simulink model "MATLAB_TEST"  (R2019b)
settings: Solver=FixedStepDiscrete  StartTime=0  StopTime=50  FixedStep=0.0025  RelTol=1e-3
undefined symbols (not defined in the file): BCM_COM_PROC_P20, BCM_COM_PROC_P20_SFW_R2018b, BCM_COM_PROC_P2_5, BCM_COM_PROC_P2_5_SFW_R2018b, BCM_COM_PROC_P5, BCM_COM_PROC_P5_SFW_R2018b, BCMA_ACCU_PT_Conf_Flt, BCMA_ACCU_PT_Unconf_Flt, BCMA_Antiskid_Off_Sanction, BCMA_Avionics_Conf_Flt, BCMA_BCM_CCDL_Conf_Flt, BCMA_BCM_CCDL_Unconf_Flt, BCMA_BCM_DBCU_INHIBITION_Conf_Flt, BCMA_BCM_DBCU_INHIBITION_Unconf_Flt, BCMA_BCP_ALT_Disp_Sw_Conf_Flt, BCMA_BCP_ALT_Disp_Sw_Unconf_Flt, BCMA_BCP_ALT_SW_ON_CMD_Conf_Flt, BCMA_BCP_ALT_SW_ON_CMD_Unconf_Flt, BCMA_BCP_PARK_OFF_SW_CMD_Conf_Flt, BCMA_BCP_PARK_OFF_SW_CMD_Unconf_Flt, BCMA_CF_BSELV_JCL, BCMA_CF_BSELV_JOP, BCMA_CF_BSELV_OC, BCMA_CF_BSELV_SC, BCMA_CF_LH_SV_JCL, BCMA_CF_LH_SV_JOP, BCMA_CF_LH_SV_OC, BCMA_CF_LH_SV_SC, BCMA_CF_PARK_BRK, BCMA_CF_RESIDUAL_PRESS, BCMA_CF_RH_SV_JCL, BCMA_CF_RH_SV_JOP, BCMA_CF_RH_SV_OC, BCMA_CF_RH_SV_SC, BCMA_CF_SELV_JCL, BCMA_CF_SELV_JOP, BCMA_CF_SELV_OC, BCMA_CF_SELV_SC, BCMA_CF_SV_DRIFT, BCMA_DBCU_ALT_MODE_Conf_Flt, BCMA_DBCU_ALT_MODE_Unconf_Flt, BCMA_DBCU_BRK_ORDER_FAIL_Conf_Flt, BCMA_DBCU_BRK_ORDER_FAIL_Unconf_Flt, BCMA_DBCU_Conf_Flt, BCMA_DBCU_DISPATCH_SW_ON_Conf_Flt, BCMA_DBCU_DISPATCH_SW_ON_Unconf_Flt, BCMA_DBCU_FAILED_Conf_Flt, BCMA_DBCU_FAILED_Unconf_Flt, BCMA_DFCS1_Capsule_Validity, BCMA_DFCS1_Label202_Corrupted, BCMA_DFCS1_Label202_Not_Refreshed, BCMA_DFCS1_Label204_Corrupted, BCMA_DFCS1_Label204_Not_Refreshed, BCMA_DFCS1_Label205_Corrupted, BCMA_DFCS1_Label205_Not_Refreshed, BCMA_DFCS1_Label206_Corrupted, BCMA_DFCS1_Label206_Not_Refreshed, BCMA_DFCS1_Label207_Corrupted, BCMA_DFCS1_Label207_Not_Refreshed, BCMA_DFCS3_Capsule_Validity ... (+762)
libraries: simulink x73, lib_MBD_Control x5
(part 15 of 16)

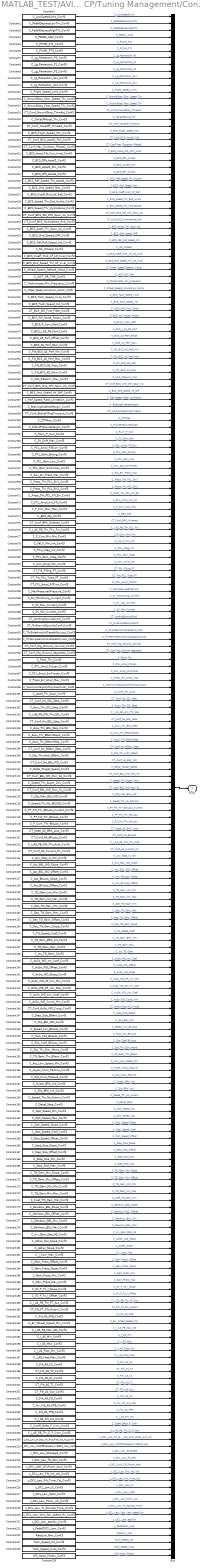
== system MATLAB_TEST/AVIONICS/Brake_Control_Module_Side_A/BCSA Controller CP/Tuning Management/Conf3 ==
  Bus : BusCreator  Inputs=226
  Constant1 : Constant  Value=C_LowSpeedLimit_Conf3
  Constant10 : Constant  Value=C_Lg_Retraction_SL1_Conf3
  Constant100 : Constant  Value=C_Accel_Thr_Auso_Conf3
  Constant101 : Constant  Value=CT_Conf_No_SSL_Step_Conf3
  Constant102 : Constant  Value=C_Accu_Thr_SSL_Step_Conf3
  Constant103 : Constant  Value=C_I_AS_PB_OW_Thr_SSL_Conf3
  Constant104 : Constant  Value=CT_Conf_No_BSL_Step_Conf3
  Constant105 : Constant  Value=C_Accu_Thr_BSL_Step_Conf3
  Constant106 : Constant  Value=C_Accu_Thr_BGamStep0_Conf3
  Constant107 : Constant  Value=C_Accu_Thr_BGamStep_Conf3
  Constant108 : Constant  Value=CT_Conf_No_BGam_Step_Conf3
  Constant109 : Constant  Value=C_Slip_Thr_Auth_BGam_Conf3
  Constant11 : Constant  Value=C_Lg_Retraction_SL2_Conf3
  Constant110 : Constant  Value=CT_Conf_No_BSL_WD_Conf3
  Constant111 : Constant  Value=C_Delta_Target_Speed_Conf3
  Constant112 : Constant  Value=CT_Conf_BSL_WD_Mon_FA_Conf3
  Constant113 : Constant  Value=C_Speed_Thr_Augm_Dim_Conf3
  Constant114 : Constant  Value=CT_Conf_BSL_WD_Mon_SL_Conf3
  Constant115 : Constant  Value=C_Slip_Max_BSL_WD_Conf3
  Constant116 : Constant  Value=C_Speed_Thr_No_BSLWD_Conf3
  Constant117 : Constant  Value=C_PT_Filt_Thr_BKLoss_Current_Conf3
  Constant118 : Constant  Value=C_PT_Filt_Thr_BKLoss_Conf3
  Constant119 : Constant  Value=C_P_Com_Thr_BKLoss_Conf3
  Constant12 : Constant  Value=C_Flight_Speed_Limit_Conf3
  Constant120 : Constant  Value=CT_Keep_AS_BRK_Loss_Conf3
  Constant121 : Constant  Value=CT_Conf_AS_BKLoss_Conf3
  Constant122 : Constant  Value=C_I_AS_PB_OW_Thr_Auth_Conf3
  Constant123 : Constant  Value=CT_Conf_AS_Current_On_Conf3
  Constant124 : Constant  Value=C_Any_Step_In_Min_Conf3
  Constant125 : Constant  Value=C_Acc_BSL_WD_Slope_Conf3
  Constant126 : Constant  Value=C_Acc_BSL_WD_Offset_Conf3
  Constant127 : Constant  Value=C_Acc_BKLoss_Slope_Conf3
  Constant128 : Constant  Value=C_Acc_BKLoss_Offset_Conf3
  Constant129 : Constant  Value=C_TG_Gam_Init_Min_Conf3
  Constant13 : Constant  Value=C_GroundStop_Slow_Speed_Thr_Conf3
  Constant130 : Constant  Value=C_TG_Gam_Init_Max_Conf3
  Constant131 : Constant  Value=C_Dec_TG_Gam_Min_Conf3
  Constant132 : Constant  Value=C_Dec_TG_Gam_Max_Conf3
  Constant133 : Constant  Value=C_Dec_TG_Gam_Offset_Conf3
  Constant134 : Constant  Value=C_Dec_TG_Gam_Slope_Conf3
  Constant135 : Constant  Value=C_TG_Speed_Coef_Conf3
  Constant136 : Constant  Value=C_TG_Gam_BRK_Init_Conf3
  Constant137 : Constant  Value=C_TG_Gam_Max_Conf3
  Constant138 : Constant  Value=C_Inc_TG_Gam_Conf3
  Constant139 : Constant  Value=C_AuSo_WD_Inc_Coef_Conf3
  Constant14 : Constant  Value=C_GroundStop_Fast_Speed_Thr_Conf3
  Constant140 : Constant  Value=C_AuSo_WD_Offset_Conf3
  Constant141 : Constant  Value=C_AuSo_WD_Slope_Conf3
  Constant142 : Constant  Value=C_AuSo_WD_SP_Lim_Min_Conf3
  Constant143 : Constant  Value=C_AuSo_WD_SP_Lim_Max_Conf3
  Constant144 : Constant  Value=C_AuSo_WD_Lim_Coef_Conf3
  Constant145 : Constant  Value=C_AuSo_WD_Count_Min_Conf3
  Constant146 : Constant  Value=CT_Conf_AuSo_WD_Froze_Conf3
  Constant147 : Constant  Value=C_Step_Size_BGam_Conf3
  Constant148 : Constant  Value=C_Slip_BSL_WD_Conf3
  Constant149 : Constant  Value=C_Speed_Lim_BKLoss_Conf3
  Constant15 : Constant  Value=CT_Conf_GroundStop_TimeAct_Conf3
  Constant150 : Constant  Value=C_Tach_Fail_BKLoss_Conf3
  Constant151 : Constant  Value=C_Slip_Coef_BKLoss_Conf3
  Constant152 : Constant  Value=C_Slip_Thr_Dim_Maint_Conf3
  Constant153 : Constant  Value=C_TG_Gam_Thr_BGam_Conf3
  Constant154 : Constant  Value=C_Acc_Low_Speed_Min_Conf3
  Constant155 : Constant  Value=C_Hyper_Cons_Passive_Conf3
  Constant156 : Constant  Value=C_Slip_Cons_Passive_Conf3
  Constant157 : Constant  Value=C_Hyper_BRK_Init_Conf3
  Constant158 : Constant  Value=C_Slip_BRK_Init_Conf3
  Constant159 : Constant  Value=C_Speed_Thr_No_Autom_Conf3
  Constant16 : Constant  Value=C_TakeOffAccel_Thr_Conf3
  Constant160 : Constant  Value=C_Decel_Step_Conf3
  Constant161 : Constant  Value=C_Opti_Speed_Min_Conf3
  Constant162 : Constant  Value=C_Opti_Speed_Max_Conf3
  Constant163 : Constant  Value=C_Opti_Speed_Slope_Conf3
  Constant164 : Constant  Value=C_Opti_Speed_Coef_Conf3
  Constant165 : Constant  Value=C_Opti_Speed_Offset_Conf3
  Constant166 : Constant  Value=C_Step_Size_Slope_Conf3
  Constant167 : Constant  Value=C_Step_Size_Offset_Conf3
  Constant168 : Constant  Value=C_Step_Size_Min_Conf3
  Constant169 : Constant  Value=C_Step_Size_Max_Conf3
  Constant17 : Constant  Value=CT_Conf_TakeOff_TimeAct_Conf3
  Constant170 : Constant  Value=C_TG_Gam_Min_Slope_Conf3
  Constant171 : Constant  Value=C_TG_Gam_Min_Offset_Conf3
  Constant172 : Constant  Value=C_TG_Gam_Min_Min_Conf3
  Constant173 : Constant  Value=C_TG_Gam_Min_Max_Conf3
  Constant174 : Constant  Value=C_Coef_TG_Gam_Min_Conf3
  Constant175 : Constant  Value=C_DenAccu_BSL_Slope_Conf3
  Constant176 : Constant  Value=C_DenAccu_BSL_Offset_Conf3
  Constant177 : Constant  Value=C_DenAccu_BSL_Min_Conf3
  Constant178 : Constant  Value=C_DenAccu_BSL_Max_Conf3
  Constant179 : Constant  Value=C_Inv_Gain_Stat_AS_Conf3
  Constant18 : Constant  Value=C_BCS_Flight_Speed_Min_Conf3
  Constant180 : Constant  Value=C_Adher_Opt_Slope_Conf3
  Constant181 : Constant  Value=C_Adher_Slope_Conf3
  Constant182 : Constant  Value=C_I_Com_Max_Conf3
  Constant183 : Constant  Value=C_Gain_Press_Offset_Conf3
  Constant184 : Constant  Value=C_Gain_Press_Slope_Conf3
  Constant185 : Constant  Value=C_Gain_Press_Min_Conf3
  Constant186 : Constant  Value=C_Gain_Press_Max_Conf3
  Constant187 : Constant  Value=C_SV_P_To_I_Slope_Conf3
  Constant188 : Constant  Value=C_SV_P_To_I_Offset_Conf3
  Constant189 : Constant  Value=C_I_AS_PB_Thr_PT_Aut_Conf3
  Constant19 : Constant  Value=CT_Conf_BCS_Accel2_Fail_Conf3
  Constant190 : Constant  Value=CT_Filt_PT_Filt_Autom_Conf3
  Constant191 : Constant  Value=C_Filt_AS_KPB_Conf3
  Constant192 : Constant  Value=C_Err_Wheel_Speed_Min_Conf3
  Constant193 : Constant  Value=C_I_AS_PB_Max_ND_Conf3
  Constant194 : Constant  Value=C_I_AS_Min_Conf3
  Constant195 : Constant  Value=C_I_AS_Max_Conf3
  Constant196 : Constant  Value=C_I_AS_Fast_Min_Conf3
  Constant197 : Constant  Value=C_I_AS_Fast_Max_Conf3
  Constant198 : Constant  Value=C_Filt_AS_K2_Conf3
  Constant199 : Constant  Value=CT_Filt_AS_T2_Conf3
  Constant2 : Constant  Value=C_PedalDepressLowThr_Conf3
  Constant20 : Constant  Value=CT_Conf_Max_Duration_Phase2_Conf3
  Constant200 : Constant  Value=C_Filt_AS_K1_Conf3
  Constant201 : Constant  Value=CT_Filt_AS_T1_Conf3
  Constant202 : Constant  Value=CT_Filt_AS_Out_Conf3
  Constant203 : Constant  Value=C_Filt_AS_K0_Conf3
  Constant204 : Constant  Value=C_Inv_Filt_AS_KPB_Conf3
  Constant205 : Constant  Value=C_Filt_AS_TPB_Conf3
  Constant206 : Constant  Value=C_I_AS_Filt_Init_Conf3
  Constant207 : Constant  Value=C_Coeff_Delta_P_Com_Conf3
  Constant208 : Constant  Value=C_I_AS_PB_Thr_D_P_Com_Conf3
  Constant209 : Constant  Value=c_DCL_Law_CT_BCS_WS_First_Filter_Acc_AC_Conf3
  Constant21 : Constant  Value=C_BCS_Accel_Filt_Corr_Inval_Conf3
  Constant210 : Constant  Value=c_DCL_Law_CutOffFrequencyVSGRS_Law_Conf3
  Constant211 : Constant  Value=c_DCL_Law_Strategie_Conf3
  Constant212 : Constant  Value=c_DCL_Law_filt_8Hz_Conf3
  Constant213 : Constant  Value=c_DCL_LAW_DCLPcom_bool_Conf3
  Constant214 : Constant  Value=c_DCL_Law_Filt_Init_Val_Conf3
  Constant215 : Constant  Value=c_DCL_Law_Filt_Time_Cst_Conf3
  Constant216 : Constant  Value=c_DCL_Law_Ki_Conf3
  Constant217 : Constant  Value=c_DCL_Law_Kpb2_Conf3
  Constant218 : Constant  Value=c_DCL_Law_Pcom_var_Conf3
  Constant219 : Constant  Value=c_DCL_Law_Ts_Sample_Time_Conf3
  Constant22 : Constant  Value=C_BCS_Dflt_Accel2_Conf3
  Constant220 : Constant  Value=c_DCL_Law_Very_law_speed_thr_Conf3
  Constant221 : Constant  Value=c_DCL_Law_epsilon_Conf3
  Constant222 : Constant  Value=c_Pedal2DCL_Law_Conf3
  Constant223 : Constant  Value=RateLim_Max_Conf3
  Constant224 : Constant  Value=Tach_Speed_Init_Conf3
  Constant225 : Constant  Value=Tach_Speed_Inval_Conf3
  Constant226 : Constant  Value=WS_Noise_Factor_Conf3
  Constant23 : Constant  Value=C_BCS_Accel3_Min_Conf3
  Constant24 : Constant  Value=C_BCS_Dflt_Accel4_Conf3
  Constant25 : Constant  Value=C_BCS_Ref_Speed_Thr_Accel4_Conf3
  Constant26 : Constant  Value=C_BCS_Gnd_Speed_Max_Conf3
  Constant27 : Constant  Value=C_BCS_Coeff_Mult_Inf_Ref_Conf3
  Constant28 : Constant  Value=C_BCS_Speed_Thr_End_Hydro_Conf3
  Constant29 : Constant  Value=C_BCS_Speed_Thr_Hydroplane_Conf3
  Constant3 : Constant  Value=C_PedalDepressHighThr_Conf3
  Constant30 : Constant  Value=CT_Conf_BCS_Gbl_Whl_Spun_Up_Conf3
  Constant31 : Constant  Value=CT_Conf_BCS_Hydroplane_End_Conf3
  Constant32 : Constant  Value=C_BCS_Accel_Thr_Spun_Up_Conf3
  Constant33 : Constant  Value=C_BCS_Gnd_Speed_Diff_Conf3
  Constant34 : Constant  Value=C_BCS_Gbl_Ref_Speed_Init_Conf3
  Constant35 : Constant  Value=C_Nb_Wheels_Conf3
  Constant36 : Constant  Value=C_BCS_Coeff_Mult_Inf_LG_Inval_Conf3
  Constant37 : Constant  Value=C_BCS_Gnd_Speed_Thr_LG_Inval_Conf3
  Constant38 : Constant  Value=C_Wheel_Speed_Default_Value_Conf3
  Constant39 : Constant  Value=C_WST_OR_THR_Conf3
  Constant4 : Constant  Value=C_PEDAL_LAW_Conf3
  Constant40 : Constant  Value=C_Tachometer_Min_Frequency_Conf3
  Constant41 : Constant  Value=C_Wheel_Speed_Conversion_Factor_Conf3
  Constant42 : Constant  Value=C_BCS_Tach_Speed_Inval_Conf3
  Constant43 : Constant  Value=C_BCS_Tach_Speed_Init_Conf3
  Constant44 : Constant  Value=CT_BCS_WS_First_Filter_Conf3
  Constant45 : Constant  Value=C_BCS_WS_Noise_Factor_Conf3
  Constant46 : Constant  Value=C_BCS_P_Com_Perf_Conf3
  Constant47 : Constant  Value=C_BCS_I_AS_PB_Perf_Conf3
  Constant48 : Constant  Value=C_BCS_AS_Perf_Offset_Conf3
  Constant49 : Constant  Value=C_BCS_AS_Perf_Gain_Conf3
  Constant5 : Constant  Value=C_PCOM_FT1_Conf3
  Constant50 : Constant  Value=C_Filt_BCS_AS_Perf_Min_Conf3
  Constant51 : Constant  Value=C_Filt_BCS_AS_Perf_Max_Conf3
  Constant52 : Constant  Value=C_Filt_BCS_AS_Fast_Conf3
  Constant53 : Constant  Value=C_Filt_BCS_AS_Slow_Conf3
  Constant54 : Constant  Value=C_Wst_RateLim_Max_Conf3
  Constant55 : Constant  Value=CT_Conf_BCS_One_Whl_Spun_Up_Conf3
  Constant56 : Constant  Value=C_BCS_Gnd_Speed_Inf_Diff_Conf3
  Constant57 : Constant  Value=C_Ref_Speed_Rate_Limitation_Conf3
  Constant58 : Constant  Value=C_BrakingOrderedMargin_Conf3
  Constant59 : Constant  Value=CT_Conf_BrakeFillingTimeout_Conf3
  Constant6 : Constant  Value=C_PCOM_FT3_Conf3
  Constant60 : Constant  Value=C_ZTPMax_Conf3
  Constant61 : Constant  Value=C_FilloutPressureMargin_Conf3
  Constant62 : Constant  Value=C_RLim_P_Corr_Conf3
  Constant63 : Constant  Value=C_SV_Drift_Max_Conf3
  Constant64 : Constant  Value=C_PCL_Ampl_FillCorr_Conf3
  Constant65 : Constant  Value=C_PCL_Gain_Strong_Conf3
  Constant66 : Constant  Value=C_PCL_Gain_Low_Conf3
  Constant67 : Constant  Value=C_PCL_Gain_SmFrozen_Conf3
  Constant68 : Constant  Value=C_Squ_Err_Press_Max_Conf3
  Constant69 : Constant  Value=C_Press_Thr_PCL_Err1_Conf3
  Constant7 : Constant  Value=C_Lg_Retraction_P0_Conf3
  Constant70 : Constant  Value=C_Press_Thr_PCL_Err2_Conf3
  Constant71 : Constant  Value=C_Press_Thr_PCL_Fill_Err_Conf3
  Constant72 : Constant  Value=C_PCL_Ampl_Init_Fill_Conf3
  Constant73 : Constant  Value=C_P_Corr_Max_Max_Conf3
  Constant74 : Constant  Value=C_BCS_Ztp_Conf3
  Constant75 : Constant  Value=CT_Conf_BRK_Ordered_Conf3
  Constant76 : Constant  Value=C_I_AS_PB_Thr_PCL_Frz_Conf3
  Constant77 : Constant  Value=C_P_Corr_Min_Min_Conf3
  Constant78 : Constant  Value=C_Val_P_Min_Init_Conf3
  Constant79 : Constant  Value=C_PCL_Integ_Init_Conf3
  Constant8 : Constant  Value=C_Lg_Retraction_P1_Conf3
  Constant80 : Constant  Value=C_PCL_Gain_Integ_Conf3
  Constant81 : Constant  Value=C_Corr_Ampl_Min_Conf3
  Constant82 : Constant  Value=CT_Filt_Filling_PT_Conf3
  Constant83 : Constant  Value=CT_Filt_PCL_Tube_PT_Conf3
  Constant84 : Constant  Value=CT_PCL_Ampl_FillCorr_Conf3
  Constant85 : Constant  Value=C_MaxMeasuredPressure_Conf3
  Constant86 : Constant  Value=C_SV_Monitoring_Current_Conf3
  Constant87 : Constant  Value=C_SV_Max_Current_Conf3
  Constant88 : Constant  Value=C_SV_Min_Current_Conf3
  Constant89 : Constant  Value=CT_LandingSpunUpConf_Conf3
  Constant9 : Constant  Value=C_Lg_Retraction_P2_Conf3
  Constant90 : Constant  Value=CT_OnGroundSpunUpConf_Conf3
  Constant91 : Constant  Value=C_ThrSideAntiskidCapabilityLoss_Conf3
  Constant92 : Constant  Value=C_ThrPerimeterAntiskidCapabilityLoss_Conf3
  Constant93 : Constant  Value=CT_Conf_Nlg_Ground_nominal_Conf3
  Constant94 : Constant  Value=CT_Conf_Nlg_Ground_degraded_Conf3
  Constant95 : Constant  Value=C_Pitch_Thr_Conf3
  Constant96 : Constant  Value=C_PCL_Ampl_Frozen_Conf3
  Constant97 : Constant  Value=C_PCL_Ampl_SmFrozen_Conf3
  Constant98 : Constant  Value=C_Press_Err_Ampl_Max_Conf3
  Constant99 : Constant  Value=C_MaximumMarginWithHydraulicLost_Conf3
  Out1 : Outport  VectorParamsAs1DForOutWhenUnconnected=off
  wires:
  Constant1/1 -> Bus/1  "C_LowSpeedLimit"
  Constant2/1 -> Bus/2  "C_PedalDepressLowThr"
  Constant3/1 -> Bus/3  "C_PedalDepressHighThr"
  Constant4/1 -> Bus/4  "C_PEDAL_LAW"
  Constant5/1 -> Bus/5  "C_PCOM_FT1"
  Constant6/1 -> Bus/6  "C_PCOM_FT3"
  Constant7/1 -> Bus/7  "C_Lg_Retraction_P0"
  Constant8/1 -> Bus/8  "C_Lg_Retraction_P1"
  Constant9/1 -> Bus/9  "C_Lg_Retraction_P2"
  Constant10/1 -> Bus/10  "C_Lg_Retraction_SL1"
  Constant11/1 -> Bus/11  "C_Lg_Retraction_SL2"
  Constant12/1 -> Bus/12  "C_Flight_Speed_Limit"
  Constant13/1 -> Bus/13  "C_GroundStop_Slow_Speed_Thr"
  Constant14/1 -> Bus/14  "C_GroundStop_Fast_Speed_Thr"
  Constant15/1 -> Bus/15  "CT_Conf_GroundStop_TimeAct"
  Constant16/1 -> Bus/16  "C_TakeOffAccel_Thr"
  Constant17/1 -> Bus/17  "CT_Conf_TakeOff_TimeAct"
  Constant18/1 -> Bus/18  "C_BCS_Flight_Speed_Min"
  Constant19/1 -> Bus/19  "CT_Conf_BCS_Accel2_Fail"
  Constant20/1 -> Bus/20  "CT_Conf_Max_Duration_Phase2"
  Constant21/1 -> Bus/21  "C_BCS_Accel_Filt_Corr_Inval"
  Constant22/1 -> Bus/22  "C_BCS_Dflt_Accel2"
  Constant23/1 -> Bus/23  "C_BCS_Accel3_Min"
  Constant24/1 -> Bus/24  "C_BCS_Dflt_Accel4"
  Constant25/1 -> Bus/25  "C_BCS_Ref_Speed_Thr_Accel4"
  Constant26/1 -> Bus/26  "C_BCS_Gnd_Speed_Max"
  Constant27/1 -> Bus/27  "C_BCS_Coeff_Mult_Inf_Ref"
  Constant28/1 -> Bus/28  "C_BCS_Speed_Thr_End_Hydro"
  Constant29/1 -> Bus/29  "C_BCS_Speed_Thr_Hydroplane"
  Constant30/1 -> Bus/30  "CT_Conf_BCS_Gbl_Whl_Spun_Up"
  Constant31/1 -> Bus/31  "CT_Conf_BCS_Hydroplane_End"
  Constant32/1 -> Bus/32  "C_BCS_Accel_Thr_Spun_Up"
  Constant33/1 -> Bus/33  "C_BCS_Gnd_Speed_Diff"
  Constant34/1 -> Bus/34  "C_BCS_Gbl_Ref_Speed_Init"
  Constant35/1 -> Bus/35  "C_Nb_Wheels"
  Constant36/1 -> Bus/36  "C_BCS_Coeff_Mult_Inf_LG_Inval"
  Constant37/1 -> Bus/37  "C_BCS_Gnd_Speed_Thr_LG_Inval"
  Constant38/1 -> Bus/38  "C_Wheel_Speed_Default_Value"
  Constant39/1 -> Bus/39  "C_WST_OR_THR"
  Constant40/1 -> Bus/40  "C_Tachometer_Min_Frequency"
  Constant41/1 -> Bus/41  "C_Wheel_Speed_Conversion_Factor"
  Constant42/1 -> Bus/42  "C_BCS_Tach_Speed_Inval"
  Constant43/1 -> Bus/43  "C_BCS_Tach_Speed_Init"
  Constant44/1 -> Bus/44  "CT_BCS_WS_First_Filter"
  Constant45/1 -> Bus/45  "C_BCS_WS_Noise_Factor"
  Constant46/1 -> Bus/46  "C_BCS_P_Com_Perf"
  Constant47/1 -> Bus/47  "C_BCS_I_AS_PB_Perf"
  Constant48/1 -> Bus/48  "C_BCS_AS_Perf_Offset"
  Constant49/1 -> Bus/49  "C_BCS_AS_Perf_Gain"
  Constant50/1 -> Bus/50  "C_Filt_BCS_AS_Perf_Min"
  Constant51/1 -> Bus/51  "C_Filt_BCS_AS_Perf_Max"
  Constant52/1 -> Bus/52  "C_Filt_BCS_AS_Fast"
  Constant53/1 -> Bus/53  "C_Filt_BCS_AS_Slow"
  Constant54/1 -> Bus/54  "C_Wst_RateLim_Max"
  Constant55/1 -> Bus/55  "CT_Conf_BCS_One_Whl_Spun_Up"
  Constant56/1 -> Bus/56  "C_BCS_Gnd_Speed_Inf_Diff"
  Constant57/1 -> Bus/57  "C_Ref_Speed_Rate_Limitation"
  Constant58/1 -> Bus/58  "C_BrakingOrderedMargin"
  Constant59/1 -> Bus/59  "CT_Conf_BrakeFillingTimeout"
  Constant60/1 -> Bus/60  "C_ZTPMax"
  Constant61/1 -> Bus/61  "C_FilloutPressureMargin"
  Constant62/1 -> Bus/62  "C_RLim_P_Corr"
  Constant63/1 -> Bus/63  "C_SV_Drift_Max"
  Constant64/1 -> Bus/64  "C_PCL_Ampl_FillCorr"
  Constant65/1 -> Bus/65  "C_PCL_Gain_Strong"
  Constant66/1 -> Bus/66  "C_PCL_Gain_Low"
  Constant67/1 -> Bus/67  "C_PCL_Gain_SmFrozen"
  Constant68/1 -> Bus/68  "C_Squ_Err_Press_Max"
  Constant69/1 -> Bus/69  "C_Press_Thr_PCL_Err1"
  Constant70/1 -> Bus/70  "C_Press_Thr_PCL_Err2"
  Constant71/1 -> Bus/71  "C_Press_Thr_PCL_Fill_Err"
  Constant72/1 -> Bus/72  "C_PCL_Ampl_Init_Fill"
  Constant73/1 -> Bus/73  "C_P_Corr_Max_Max"
  Constant74/1 -> Bus/74  "C_BCS_Ztp"
  Constant75/1 -> Bus/75  "CT_Conf_BRK_Ordered"
  Constant76/1 -> Bus/76  "C_I_AS_PB_Thr_PCL_Frz"
  Constant77/1 -> Bus/77  "C_P_Corr_Min_Min"
  Constant78/1 -> Bus/78  "C_Val_P_Min_Init"
  Constant79/1 -> Bus/79  "C_PCL_Integ_Init"
  Constant80/1 -> Bus/80  "C_PCL_Gain_Integ"
  Constant81/1 -> Bus/81  "C_Corr_Ampl_Min"
  Constant82/1 -> Bus/82  "CT_Filt_Filling_PT"
  Constant83/1 -> Bus/83  "CT_Filt_PCL_Tube_PT"
  Constant84/1 -> Bus/84  "CT_PCL_Ampl_FillCorr"
  Constant85/1 -> Bus/85  "C_MaxMeasuredPressure"
  Constant86/1 -> Bus/86  "C_SV_Monitoring_Current"
  Constant87/1 -> Bus/87  "C_SV_Max_Current"
  Constant88/1 -> Bus/88  "C_SV_Min_Current"
  Constant89/1 -> Bus/89  "CT_LandingSpunUpConf"
  Constant90/1 -> Bus/90  "CT_OnGroundSpunUpConf"
  Constant91/1 -> Bus/91  "C_ThrSideAntiskidCapabilityLoss"
  Constant92/1 -> Bus/92  "C_ThrPerimeterAntiskidCapabilityLoss"
  Constant93/1 -> Bus/93  "CT_Conf_Nlg_Ground_nominal"
  Constant94/1 -> Bus/94  "CT_Conf_Nlg_Ground_degraded"
  Constant95/1 -> Bus/95  "C_Pitch_Thr"
  Constant96/1 -> Bus/96  "C_PCL_Ampl_Frozen"
  Constant97/1 -> Bus/97  "C_PCL_Ampl_SmFrozen"
  Constant98/1 -> Bus/98  "C_Press_Err_Ampl_Max"
  Constant99/1 -> Bus/99  "C_MaximumMarginWithHydraulicLost"
  Constant100/1 -> Bus/100  "C_Accel_Thr_Auso"
  Constant101/1 -> Bus/101  "CT_Conf_No_SSL_Step"
  Constant102/1 -> Bus/102  "C_Accu_Thr_SSL_Step"
  Constant103/1 -> Bus/103  "C_I_AS_PB_OW_Thr_SSL"
  Constant104/1 -> Bus/104  "CT_Conf_No_BSL_Step"
  Constant105/1 -> Bus/105  "C_Accu_Thr_BSL_Step"
  Constant106/1 -> Bus/106  "C_Accu_Thr_BGamStep0"
  Constant107/1 -> Bus/107  "C_Accu_Thr_BGamStep"
  Constant108/1 -> Bus/108  "CT_Conf_No_BGam_Step"
  Constant109/1 -> Bus/109  "C_Slip_Thr_Auth_BGam"
  Constant110/1 -> Bus/110  "CT_Conf_No_BSL_WD"
  Constant111/1 -> Bus/111  "C_Delta_Target_Speed"
  Constant112/1 -> Bus/112  "CT_Conf_BSL_WD_Mon_FA"
  Constant113/1 -> Bus/113  "C_Speed_Thr_Augm_Dim"
  Constant114/1 -> Bus/114  "CT_Conf_BSL_WD_Mon_SL"
  Constant115/1 -> Bus/115  "C_Slip_Max_BSL_WD"
  Constant116/1 -> Bus/116  "C_Speed_Thr_No_BSLWD"
  Constant117/1 -> Bus/117  "C_PT_Filt_Thr_BKLoss_Current"
  Constant118/1 -> Bus/118  "C_PT_Filt_Thr_BKLoss"
  Constant119/1 -> Bus/119  "C_P_Com_Thr_BKLoss"
  Constant120/1 -> Bus/120  "CT_Keep_AS_BRK_Loss"
  Constant121/1 -> Bus/121  "CT_Conf_AS_BKLoss"
  Constant122/1 -> Bus/122  "C_I_AS_PB_OW_Thr_Auth"
  Constant123/1 -> Bus/123  "CT_Conf_AS_Current_On"
  Constant124/1 -> Bus/124  "C_Any_Step_In_Min"
  Constant125/1 -> Bus/125  "C_Acc_BSL_WD_Slope"
  Constant126/1 -> Bus/126  "C_Acc_BSL_WD_Offset"
  Constant127/1 -> Bus/127  "C_Acc_BKLoss_Slope"
  Constant128/1 -> Bus/128  "C_Acc_BKLoss_Offset"
  Constant129/1 -> Bus/129  "C_TG_Gam_Init_Min"
  Constant130/1 -> Bus/130  "C_TG_Gam_Init_Max"
  Constant131/1 -> Bus/131  "C_Dec_TG_Gam_Min"
  Constant132/1 -> Bus/132  "C_Dec_TG_Gam_Max"
  Constant133/1 -> Bus/133  "C_Dec_TG_Gam_Offset"
  Constant134/1 -> Bus/134  "C_Dec_TG_Gam_Slope"
  Constant135/1 -> Bus/135  "C_TG_Speed_Coef"
  Constant136/1 -> Bus/136  "C_TG_Gam_BRK_Init"
  Constant137/1 -> Bus/137  "C_TG_Gam_Max"
  Constant138/1 -> Bus/138  "C_Inc_TG_Gam"
  Constant139/1 -> Bus/139  "C_AuSo_WD_Inc_Coef"
  Constant140/1 -> Bus/140  "C_AuSo_WD_Offset"
  Constant141/1 -> Bus/141  "C_AuSo_WD_Slope"
  Constant142/1 -> Bus/142  "C_AuSo_WD_SP_Lim_Min"
  Constant143/1 -> Bus/143  "C_AuSo_WD_SP_Lim_Max"
  Constant144/1 -> Bus/144  "C_AuSo_WD_Lim_Coef"
  Constant145/1 -> Bus/145  "C_AuSo_WD_Count_Min"
  Constant146/1 -> Bus/146  "CT_Conf_AuSo_WD_Froze"
  Constant147/1 -> Bus/147  "C_Step_Size_BGam"
  Constant148/1 -> Bus/148  "C_Slip_BSL_WD"
  Constant149/1 -> Bus/149  "C_Speed_Lim_BKLoss"
  Constant150/1 -> Bus/150  "C_Tach_Fail_BKLoss"
  Constant151/1 -> Bus/151  "C_Slip_Coef_BKLoss"
  Constant152/1 -> Bus/152  "C_Slip_Thr_Dim_Maint"
  Constant153/1 -> Bus/153  "C_TG_Gam_Thr_BGam"
  Constant154/1 -> Bus/154  "C_Acc_Low_Speed_Min"
  Constant155/1 -> Bus/155  "C_Hyper_Cons_Passive"
  Constant156/1 -> Bus/156  "C_Slip_Cons_Passive"
  Constant157/1 -> Bus/157  "C_Hyper_BRK_Init"
  Constant158/1 -> Bus/158  "C_Slip_BRK_Init"
  Constant159/1 -> Bus/159  "C_Speed_Thr_No_Autom"
  Constant160/1 -> Bus/160  "C_Decel_Step"
  Constant161/1 -> Bus/161  "C_Opti_Speed_Min"
  Constant162/1 -> Bus/162  "C_Opti_Speed_Max"
  Constant163/1 -> Bus/163  "C_Opti_Speed_Slope"
  Constant164/1 -> Bus/164  "C_Opti_Speed_Coef"
  Constant165/1 -> Bus/165  "C_Opti_Speed_Offset"
  Constant166/1 -> Bus/166  "C_Step_Size_Slope"
  Constant167/1 -> Bus/167  "C_Step_Size_Offset"
  Constant168/1 -> Bus/168  "C_Step_Size_Min"
  Constant169/1 -> Bus/169  "C_Step_Size_Max"
  Constant170/1 -> Bus/170  "C_TG_Gam_Min_Slope"
  Constant171/1 -> Bus/171  "C_TG_Gam_Min_Offset"
  Constant172/1 -> Bus/172  "C_TG_Gam_Min_Min"
  Constant173/1 -> Bus/173  "C_TG_Gam_Min_Max"
  Constant174/1 -> Bus/174  "C_Coef_TG_Gam_Min"
  Constant175/1 -> Bus/175  "C_DenAccu_BSL_Slope"
  Constant176/1 -> Bus/176  "C_DenAccu_BSL_Offset"
  Constant177/1 -> Bus/177  "C_DenAccu_BSL_Min"
  Constant178/1 -> Bus/178  "C_DenAccu_BSL_Max"
  Constant179/1 -> Bus/179  "C_Inv_Gain_Stat_AS"
  Constant180/1 -> Bus/180  "C_Adher_Opt_Slope"
  Constant181/1 -> Bus/181  "C_Adher_Slope"
  Constant182/1 -> Bus/182  "C_I_Com_Max"
  Constant183/1 -> Bus/183  "C_Gain_Press_Offset"
  Constant184/1 -> Bus/184  "C_Gain_Press_Slope"
  Constant185/1 -> Bus/185  "C_Gain_Press_Min"
  Constant186/1 -> Bus/186  "C_Gain_Press_Max"
  Constant187/1 -> Bus/187  "C_SV_P_To_I_Slope"
  Constant188/1 -> Bus/188  "C_SV_P_To_I_Offset"
  Constant189/1 -> Bus/189  "C_I_AS_PB_Thr_PT_Aut"
  Constant190/1 -> Bus/190  "CT_Filt_PT_Filt_Autom"
  Constant191/1 -> Bus/191  "C_Filt_AS_KPB"
  Constant192/1 -> Bus/192  "C_Err_Wheel_Speed_Min"
  Constant193/1 -> Bus/193  "C_I_AS_PB_Max_ND"
  Constant194/1 -> Bus/194  "C_I_AS_Min"
  Constant195/1 -> Bus/195  "C_I_AS_Max"
  Constant196/1 -> Bus/196  "C_I_AS_Fast_Min"
  Constant197/1 -> Bus/197  "C_I_AS_Fast_Max"
  Constant198/1 -> Bus/198  "C_Filt_AS_K2"
  Constant199/1 -> Bus/199  "CT_Filt_AS_T2"
  Constant200/1 -> Bus/200  "C_Filt_AS_K1"
  Constant201/1 -> Bus/201  "CT_Filt_AS_T1"
  Constant202/1 -> Bus/202  "CT_Filt_AS_Out"
  Constant203/1 -> Bus/203  "C_Filt_AS_K0"
  Constant204/1 -> Bus/204  "C_Inv_Filt_AS_KPB"
  Constant205/1 -> Bus/205  "C_Filt_AS_TPB"
  Constant206/1 -> Bus/206  "C_I_AS_Filt_Init"
  Constant207/1 -> Bus/207  "C_Coeff_Delta_P_Com"
  Constant208/1 -> Bus/208  "C_I_AS_PB_Thr_D_P_Com"
  Constant209/1 -> Bus/209  "c_DCL_Law_CT_BCS_WS_First_Filter_Acc_AC"
  Constant210/1 -> Bus/210  "c_DCL_Law_CutOffFrequencyVSGRS_Law"
  Constant211/1 -> Bus/211  "c_DCL_Law_Strategie"
  Constant212/1 -> Bus/212  "c_DCL_Law_filt_8Hz"
  Constant213/1 -> Bus/213  "c_DCL_LAW_DCLPcom_bool"
  Constant214/1 -> Bus/214  "c_DCL_Law_Filt_Init_Val"
  Constant215/1 -> Bus/215  "c_DCL_Law_Filt_Time_Cst"
  Constant216/1 -> Bus/216  "c_DCL_Law_Ki"
  Constant217/1 -> Bus/217  "c_DCL_Law_Kpb2"
  Constant218/1 -> Bus/218  "c_DCL_Law_Pcom_var"
  Constant219/1 -> Bus/219  "c_DCL_Law_Ts_Sample_Time"
  Constant220/1 -> Bus/220  "c_DCL_Law_Very_law_speed_thr"
  Constant221/1 -> Bus/221  "c_DCL_Law_epsilon"
  Constant222/1 -> Bus/222  "c_Pedal2DCL_Law"
  Constant223/1 -> Bus/223  "RateLim_Max"
  Constant224/1 -> Bus/224  "Tach_Speed_Init"
  Constant225/1 -> Bus/225  "Tach_Speed_Inval"
  Constant226/1 -> Bus/226  "WS_Noise_Factor"
  Bus/1 -> Out1/1

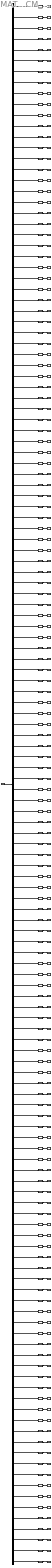
== system MATLAB_TEST/AVIONICS/Brake_Control_Module_Side_A/BCSA Controller CP/BCM_COM_PROC_P20/BCM_COM_PROC_P20/Subsystem ==
  In1 : Inport
  BusSelector : BusSelector  OutputSignals=CT_Conf_AS_BKLoss,CT_Conf_AS_Current_On,CT_Conf_AuSo_WD_Froze,CT_Conf_BCS_Accel2_Fail,CT_Conf_BCS_Gbl_Whl_Spun_Up,CT_Conf_BCS_Hydroplane_End,CT_Conf_BCS_One_Whl_Spun_Up,CT_Conf_BSL_WD_Mon_FA,CT_Conf_BSL_WD_Mon_SL,CT_Conf_BrakeFillingTimeout,CT_Conf_GroundStop_TimeAct,CT_Conf_Max_Duration_Phase2,CT_Conf_Nlg_Ground_degraded,CT_Conf_Nlg_Ground_nominal,CT_Conf_No_BGam_Step,CT_Conf_No_BSL_Step,CT_Conf_No_BSL_WD,CT_Conf_No_SSL_Step,CT_Conf_TakeOff_TimeAct,CT_Filt_PT_Filt_Autom,CT_Keep_AS_BRK_Loss,CT_LandingSpunUpConf,CT_OnGroundSpunUpConf,C_Acc_BKLoss_Offset,C_Acc_BKLoss_Slope,C_Acc_BSL_WD_Offset,C_Acc_BSL_WD_Slope,C_Acc_Low_Speed_Min,C_Accel_Thr_Auso,C_Accu_Thr_BGamStep,C_Accu_Thr_BGamStep0,C_Accu_Thr_BSL_Step,C_Accu_Thr_SSL_Step,C_Adher_Opt_Slope,C_Adher_Slope,C_Any_Step_In_Min,C_AuSo_WD_Count_Min,C_AuSo_WD_Inc_Coef,C_AuSo_WD_Lim_Coef,C_AuSo_WD_Offset,C_AuSo_WD_SP_Lim_Max,C_AuSo_WD_SP_Lim_Min,C_AuSo_WD_Slope,C_BCS_Accel3_Min,C_BCS_Accel_Filt_Corr_Inval,C_BCS_Accel_Thr_Spun_Up,C_BCS_Coeff_Mult_Inf_LG_Inval,C_BCS_Coeff_Mult_Inf_Ref,C_BCS_Dflt_Accel2,C_BCS_Dflt_Accel4,C_BCS_Flight_Speed_Min,C_BCS_Gbl_Ref_Speed_Init,C_BCS_Gnd_Speed_Diff,C_BCS_Gnd_Speed_Inf_Diff,C_BCS_Gnd_Speed_Max,C_BCS_Gnd_Speed_Thr_LG_Inval,C_BCS_Ref_Speed_Thr_Accel4,C_BCS_Speed_Thr_End_Hydro,C_BCS_Speed_Thr_Hydroplane,C_BrakingOrderedMargin,C_Coef_TG_Gam_Min,C_Dec_TG_Gam_Max,C_Dec_TG_Gam_Min,C_Dec_TG_Gam_Offset,C_Dec_TG_Gam_Slope,C_Decel_Step,C_Delta_Target_Speed,C_DenAccu_BSL_Max,C_DenAccu_BSL_Min,C_DenAccu_BSL_Offset,C_DenAccu_BSL_Slope,C_FilloutPressureMargin,C_Flight_Speed_Limit,C_Gain_Press_Max,C_Gain_Press_Min,C_Gain_Press_Offset,C_Gain_Press_Slope,C_GroundStop_Fast_Speed_Thr,C_GroundStop_Slow_Speed_Thr,C_Hyper_BRK_Init,C_Hyper_Cons_Passive,C_I_AS_PB_OW_Thr_Auth,C_I_AS_PB_OW_Thr_SSL,C_I_AS_PB_Thr_PT_Aut,C_I_Com_Max,C_Inc_TG_Gam,C_Inv_Gain_Stat_AS,C_Lg_Retraction_P0,C_Lg_Retraction_P1,C_Lg_Retraction_P2,C_Lg_Retraction_SL1,C_Lg_Retraction_SL2,C_LowSpeedLimit,C_MaximumMarginWithHydraulicLost,C_Nb_Wheels,C_Opti_Speed_Coef,C_Opti_Speed_Max,C_Opti_Speed_Min,C_Opti_Speed_Offset,C_Opti_Speed_Slope,C_PCOM_FT1,C_PCOM_FT3,C_PEDAL_LAW,C_PT_Filt_Thr_BKLoss,C_PT_Filt_Thr_BKLoss_Current,C_P_Com_Thr_BKLoss,C_PedalDepressHighThr,C_PedalDepressLowThr,C_Pitch_Thr,C_Ref_Speed_Rate_Limitation,C_SV_P_To_I_Offset,C_SV_P_To_I_Slope,C_Slip_BRK_Init,C_Slip_BSL_WD,C_Slip_Coef_BKLoss,C_Slip_Cons_Passive,C_Slip_Max_BSL_WD,C_Slip_Thr_Auth_BGam,C_Slip_Thr_Dim_Maint,C_Speed_Lim_BKLoss,C_Speed_Thr_Augm_Dim,C_Speed_Thr_No_Autom,C_Speed_Thr_No_BSLWD,C_Step_Size_BGam,C_Step_Size_Max,C_Step_Size_Min,C_Step_Size_Offset,C_Step_Size_Slope,C_TG_Gam_BRK_Init,C_TG_Gam_Init_Max,C_TG_Gam_Init_Min,C_TG_Gam_Max,C_TG_Gam_Min_Max,C_TG_Gam_Min_Min,C_TG_Gam_Min_Offset,C_TG_Gam_Min_Slope,C_TG_Gam_Thr_BGam,C_TG_Speed_Coef,C_Tach_Fail_BKLoss,C_TakeOffAccel_Thr,C_ThrPerimeterAntiskidCapabilityLoss,C_ThrSideAntiskidCapabilityLoss,C_ZTPMax,c_Pedal2DCL_Law
  DTC{230..248,250..252,262,324,370..371} (26 alike) : DataTypeConversion  OutDataTypeStr=int32  SaturateOnIntegerOverflow=on  RndMeth=Zero
  DTC{249,253..261,263..323,325..369,372..373} (118 alike) : DataTypeConversion  OutDataTypeStr=single  SaturateOnIntegerOverflow=on  RndMeth=Zero
  Out1 : Outport
  Out2 : Outport  Port=2
  Out3 : Outport  Port=3
  Out4 : Outport  Port=4
  Out5 : Outport  Port=5
  Out6 : Outport  Port=6
  Out7 : Outport  Port=7
  Out8 : Outport  Port=8
  Out9 : Outport  Port=9
  Out10 : Outport  Port=10
  Out11 : Outport  Port=11
  Out12 : Outport  Port=12
  Out13 : Outport  Port=13
  Out14 : Outport  Port=14
  Out15 : Outport  Port=15
  Out16 : Outport  Port=16
  Out17 : Outport  Port=17
  Out18 : Outport  Port=18
  Out19 : Outport  Port=19
  Out20 : Outport  Port=20
  Out21 : Outport  Port=21
  Out22 : Outport  Port=22
  Out23 : Outport  Port=23
  Out24 : Outport  Port=24
  Out25 : Outport  Port=25
  Out26 : Outport  Port=26
  Out27 : Outport  Port=27
  Out28 : Outport  Port=28
  Out29 : Outport  Port=29
  Out30 : Outport  Port=30
  Out31 : Outport  Port=31
  Out32 : Outport  Port=32
  Out33 : Outport  Port=33
  Out34 : Outport  Port=34
  Out35 : Outport  Port=35
  Out36 : Outport  Port=36
  Out37 : Outport  Port=37
  Out38 : Outport  Port=38
  Out39 : Outport  Port=39
  Out40 : Outport  Port=40
  Out41 : Outport  Port=41
  Out42 : Outport  Port=42
  Out43 : Outport  Port=43
  Out44 : Outport  Port=44
  Out45 : Outport  Port=45
  Out46 : Outport  Port=46
  Out47 : Outport  Port=47
  Out48 : Outport  Port=48
  Out49 : Outport  Port=49
  Out50 : Outport  Port=50
  Out51 : Outport  Port=51
  Out52 : Outport  Port=52
  Out53 : Outport  Port=53
  Out54 : Outport  Port=54
  Out55 : Outport  Port=55
  Out56 : Outport  Port=56
  Out57 : Outport  Port=57
  Out58 : Outport  Port=58
  Out59 : Outport  Port=59
  Out60 : Outport  Port=60
  Out61 : Outport  Port=61
  Out62 : Outport  Port=62
  Out63 : Outport  Port=63
  Out64 : Outport  Port=64
  Out65 : Outport  Port=65
  Out66 : Outport  Port=66
  Out67 : Outport  Port=67
  Out68 : Outport  Port=68
  Out69 : Outport  Port=69
  Out70 : Outport  Port=70
  Out71 : Outport  Port=71
  Out72 : Outport  Port=72
  Out73 : Outport  Port=73
  Out74 : Outport  Port=74
  Out75 : Outport  Port=75
  Out76 : Outport  Port=76
  Out77 : Outport  Port=77
  Out78 : Outport  Port=78
  Out79 : Outport  Port=79
  Out80 : Outport  Port=80
  Out81 : Outport  Port=81
  Out82 : Outport  Port=82
  Out83 : Outport  Port=83
  Out84 : Outport  Port=84
  Out85 : Outport  Port=85
  Out86 : Outport  Port=86
  Out87 : Outport  Port=87
  Out88 : Outport  Port=88
  Out89 : Outport  Port=89
  Out90 : Outport  Port=90
  Out91 : Outport  Port=91
  Out92 : Outport  Port=92
  Out93 : Outport  Port=93
  Out94 : Outport  Port=94
  Out95 : Outport  Port=95
  Out96 : Outport  Port=96
  Out97 : Outport  Port=97
  Out98 : Outport  Port=98
  Out99 : Outport  Port=99
  Out100 : Outport  Port=100
  Out101 : Outport  Port=101
  Out102 : Outport  Port=102
  Out103 : Outport  Port=103
  Out104 : Outport  Port=104
  Out105 : Outport  Port=105
  Out106 : Outport  Port=106
  Out107 : Outport  Port=107
  Out108 : Outport  Port=108
  Out109 : Outport  Port=109
  Out110 : Outport  Port=110
  Out111 : Outport  Port=111
  Out112 : Outport  Port=112
  Out113 : Outport  Port=113
  Out114 : Outport  Port=114
  Out115 : Outport  Port=115
  Out116 : Outport  Port=116
  Out117 : Outport  Port=117
  Out118 : Outport  Port=118
  Out119 : Outport  Port=119
  Out120 : Outport  Port=120
  Out121 : Outport  Port=121
  Out122 : Outport  Port=122
  Out123 : Outport  Port=123
  Out124 : Outport  Port=124
  Out125 : Outport  Port=125
  Out126 : Outport  Port=126
  Out127 : Outport  Port=127
  Out128 : Outport  Port=128
  Out129 : Outport  Port=129
  Out130 : Outport  Port=130
  Out131 : Outport  Port=131
  Out132 : Outport  Port=132
  Out133 : Outport  Port=133
  Out134 : Outport  Port=134
  Out135 : Outport  Port=135
  Out136 : Outport  Port=136
  Out137 : Outport  Port=137
  Out138 : Outport  Port=138
  Out139 : Outport  Port=139
  Out140 : Outport  Port=140
  Out141 : Outport  Port=141
  Out142 : Outport  Port=142
  Out143 : Outport  Port=143
  Out144 : Outport  Port=144
  wires:
  BusSelector/29 -> DTC258/1  "<C_Accel_Thr_Auso>"
  BusSelector/58 -> DTC287/1  "<C_BCS_Speed_Thr_End_Hydro>"
  BusSelector/73 -> DTC302/1  "<C_Flight_Speed_Limit>"
  BusSelector/89 -> DTC318/1  "<C_Lg_Retraction_P1>"
  BusSelector/94 -> DTC323/1  "<C_MaximumMarginWithHydraulicLost>"
  DTC242/1 -> Out13/1
  BusSelector/35 -> DTC264/1  "<C_Adher_Slope>"
  BusSelector/77 -> DTC306/1  "<C_Gain_Press_Slope>"
  DTC263/1 -> Out34/1
  BusSelector/42 -> DTC271/1  "<C_AuSo_WD_SP_Lim_Min>"
  DTC303/1 -> Out74/1
  DTC353/1 -> Out124/1
  DTC249/1 -> Out20/1
  BusSelector/123 -> DTC352/1  "<C_Speed_Thr_No_BSLWD>"
  DTC296/1 -> Out67/1
  BusSelector/126 -> DTC355/1  "<C_Step_Size_Min>"
  BusSelector/79 -> DTC308/1  "<C_GroundStop_Slow_Speed_Thr>"
  BusSelector/118 -> DTC347/1  "<C_Slip_Thr_Auth_BGam>"
  BusSelector/119 -> DTC348/1  "<C_Slip_Thr_Dim_Maint>"
  BusSelector/65 -> DTC294/1  "<C_Dec_TG_Gam_Slope>"
  DTC273/1 -> Out44/1
  BusSelector/36 -> DTC265/1  "<C_Any_Step_In_Min>"
  BusSelector/108 -> DTC337/1  "<C_PedalDepressLowThr>"
  BusSelector/107 -> DTC336/1  "<C_PedalDepressHighThr>"
  BusSelector/97 -> DTC326/1  "<C_Opti_Speed_Max>"
  BusSelector/49 -> DTC278/1  "<C_BCS_Dflt_Accel2>"
  BusSelector/111 -> DTC340/1  "<C_SV_P_To_I_Offset>"
  DTC250/1 -> Out21/1
  BusSelector/69 -> DTC298/1  "<C_DenAccu_BSL_Min>"
  DTC344/1 -> Out115/1
  BusSelector/31 -> DTC260/1  "<C_Accu_Thr_BGamStep0>"
  BusSelector/16 -> DTC245/1  "<CT_Conf_No_BSL_Step>"
  BusSelector/7 -> DTC236/1  "<CT_Conf_BCS_One_Whl_Spun_Up>"
  BusSelector/137 -> DTC366/1  "<C_TG_Gam_Thr_BGam>"
  DTC347/1 -> Out118/1
  BusSelector/138 -> DTC367/1  "<C_TG_Speed_Coef>"
  BusSelector/121 -> DTC350/1  "<C_Speed_Thr_Augm_Dim>"
  BusSelector/25 -> DTC254/1  "<C_Acc_BKLoss_Slope>"
  BusSelector/63 -> DTC292/1  "<C_Dec_TG_Gam_Min>"
  DTC311/1 -> Out82/1
  BusSelector/132 -> DTC361/1  "<C_TG_Gam_Max>"
  BusSelector/103 -> DTC332/1  "<C_PEDAL_LAW>"
  BusSelector/5 -> DTC234/1  "<CT_Conf_BCS_Gbl_Whl_Spun_Up>"
  DTC328/1 -> Out99/1
  DTC371/1 -> Out142/1
  BusSelector/11 -> DTC240/1  "<CT_Conf_GroundStop_TimeAct>"
  BusSelector/37 -> DTC266/1  "<C_AuSo_WD_Count_Min>"
  BusSelector/120 -> DTC349/1  "<C_Speed_Lim_BKLoss>"
  BusSelector/78 -> DTC307/1  "<C_GroundStop_Fast_Speed_Thr>"
  BusSelector/136 -> DTC365/1  "<C_TG_Gam_Min_Slope>"
  BusSelector/131 -> DTC360/1  "<C_TG_Gam_Init_Min>"
  BusSelector/139 -> DTC368/1  "<C_Tach_Fail_BKLoss>"
  BusSelector/85 -> DTC314/1  "<C_I_Com_Max>"
  DTC364/1 -> Out135/1
  BusSelector/46 -> DTC275/1  "<C_BCS_Accel_Thr_Spun_Up>"
  BusSelector/30 -> DTC259/1  "<C_Accu_Thr_BGamStep>"
  BusSelector/57 -> DTC286/1  "<C_BCS_Ref_Speed_Thr_Accel4>"
  BusSelector/141 -> DTC370/1  "<C_ThrPerimeterAntiskidCapabilityLoss>"
  DTC246/1 -> Out17/1
  DTC330/1 -> Out101/1
  DTC352/1 -> Out123/1
  BusSelector/113 -> DTC342/1  "<C_Slip_BRK_Init>"
  DTC361/1 -> Out132/1
  BusSelector/143 -> DTC372/1  "<C_ZTPMax>"
  BusSelector/105 -> DTC334/1  "<C_PT_Filt_Thr_BKLoss_Current>"
  BusSelector/33 -> DTC262/1  "<C_Accu_Thr_SSL_Step>"
  BusSelector/133 -> DTC362/1  "<C_TG_Gam_Min_Max>"
  BusSelector/124 -> DTC353/1  "<C_Step_Size_BGam>"
  BusSelector/130 -> DTC359/1  "<C_TG_Gam_Init_Max>"
  DTC350/1 -> Out121/1
  BusSelector/125 -> DTC354/1  "<C_Step_Size_Max>"
  BusSelector/56 -> DTC285/1  "<C_BCS_Gnd_Speed_Thr_LG_Inval>"
  DTC260/1 -> Out31/1
  BusSelector/47 -> DTC276/1  "<C_BCS_Coeff_Mult_Inf_LG_Inval>"
  DTC345/1 -> Out116/1
  DTC340/1 -> Out111/1
  BusSelector/109 -> DTC338/1  "<C_Pitch_Thr>"
  BusSelector/102 -> DTC331/1  "<C_PCOM_FT3>"
  BusSelector/92 -> DTC321/1  "<C_Lg_Retraction_SL2>"
  BusSelector/13 -> DTC242/1  "<CT_Conf_Nlg_Ground_degraded>"
  DTC339/1 -> Out110/1
  BusSelector/101 -> DTC330/1  "<C_PCOM_FT1>"
  BusSelector/144 -> DTC373/1  "<c_Pedal2DCL_Law>"
  DTC329/1 -> Out100/1
  BusSelector/71 -> DTC300/1  "<C_DenAccu_BSL_Slope>"
  BusSelector/84 -> DTC313/1  "<C_I_AS_PB_Thr_PT_Aut>"
  BusSelector/76 -> DTC305/1  "<C_Gain_Press_Offset>"
  DTC257/1 -> Out28/1
  BusSelector/80 -> DTC309/1  "<C_Hyper_BRK_Init>"
  BusSelector/66 -> DTC295/1  "<C_Decel_Step>"
  BusSelector/114 -> DTC343/1  "<C_Slip_BSL_WD>"
  DTC358/1 -> Out129/1
  BusSelector/38 -> DTC267/1  "<C_AuSo_WD_Inc_Coef>"
  BusSelector/54 -> DTC283/1  "<C_BCS_Gnd_Speed_Inf_Diff>"
  BusSelector/93 -> DTC322/1  "<C_LowSpeedLimit>"
  BusSelector/64 -> DTC293/1  "<C_Dec_TG_Gam_Offset>"
  BusSelector/53 -> DTC282/1  "<C_BCS_Gnd_Speed_Diff>"
  DTC284/1 -> Out55/1
  BusSelector/59 -> DTC288/1  "<C_BCS_Speed_Thr_Hydroplane>"
  BusSelector/129 -> DTC358/1  "<C_TG_Gam_BRK_Init>"
  BusSelector/41 -> DTC270/1  "<C_AuSo_WD_SP_Lim_Max>"
  BusSelector/26 -> DTC255/1  "<C_Acc_BSL_WD_Offset>"
  BusSelector/32 -> DTC261/1  "<C_Accu_Thr_BSL_Step>"
  DTC278/1 -> Out49/1
  DTC238/1 -> Out9/1
  BusSelector/19 -> DTC248/1  "<CT_Conf_TakeOff_TimeAct>"
  BusSelector/3 -> DTC232/1  "<CT_Conf_AuSo_WD_Froze>"
  BusSelector/6 -> DTC235/1  "<CT_Conf_BCS_Hydroplane_End>"
  BusSelector/1 -> DTC230/1  "<CT_Conf_AS_BKLoss>"
  BusSelector/91 -> DTC320/1  "<C_Lg_Retraction_SL1>"
  DTC334/1 -> Out105/1
  BusSelector/81 -> DTC310/1  "<C_Hyper_Cons_Passive>"
  DTC373/1 -> Out144/1
  DTC233/1 -> Out4/1
  BusSelector/98 -> DTC327/1  "<C_Opti_Speed_Min>"
  DTC343/1 -> Out114/1
  BusSelector/70 -> DTC299/1  "<C_DenAccu_BSL_Offset>"
  BusSelector/45 -> DTC274/1  "<C_BCS_Accel_Filt_Corr_Inval>"
  BusSelector/28 -> DTC257/1  "<C_Acc_Low_Speed_Min>"
  BusSelector/83 -> DTC312/1  "<C_I_AS_PB_OW_Thr_SSL>"
  BusSelector/142 -> DTC371/1  "<C_ThrSideAntiskidCapabilityLoss>"
  DTC294/1 -> Out65/1
  DTC310/1 -> Out81/1
  BusSelector/27 -> DTC256/1  "<C_Acc_BSL_WD_Slope>"
  BusSelector/40 -> DTC269/1  "<C_AuSo_WD_Offset>"
  BusSelector/128 -> DTC357/1  "<C_Step_Size_Slope>"
  BusSelector/18 -> DTC247/1  "<CT_Conf_No_SSL_Step>"
  BusSelector/23 -> DTC252/1  "<CT_OnGroundSpunUpConf>"
  BusSelector/39 -> DTC268/1  "<C_AuSo_WD_Lim_Coef>"
  BusSelector/55 -> DTC284/1  "<C_BCS_Gnd_Speed_Max>"
  DTC285/1 -> Out56/1
  BusSelector/88 -> DTC317/1  "<C_Lg_Retraction_P0>"
  DTC286/1 -> Out57/1
  DTC337/1 -> Out108/1
  BusSelector/86 -> DTC315/1  "<C_Inc_TG_Gam>"
  BusSelector/21 -> DTC250/1  "<CT_Keep_AS_BRK_Loss>"
  DTC270/1 -> Out41/1
  BusSelector/104 -> DTC333/1  "<C_PT_Filt_Thr_BKLoss>"
  BusSelector/116 -> DTC345/1  "<C_Slip_Cons_Passive>"
  BusSelector/2 -> DTC231/1  "<CT_Conf_AS_Current_On>"
  BusSelector/43 -> DTC272/1  "<C_AuSo_WD_Slope>"
  BusSelector/122 -> DTC351/1  "<C_Speed_Thr_No_Autom>"
  DTC360/1 -> Out131/1
  BusSelector/90 -> DTC319/1  "<C_Lg_Retraction_P2>"
  BusSelector/134 -> DTC363/1  "<C_TG_Gam_Min_Min>"
  BusSelector/95 -> DTC324/1  "<C_Nb_Wheels>"
  BusSelector/99 -> DTC328/1  "<C_Opti_Speed_Offset>"
  BusSelector/110 -> DTC339/1  "<C_Ref_Speed_Rate_Limitation>"
  BusSelector/44 -> DTC273/1  "<C_BCS_Accel3_Min>"
  BusSelector/100 -> DTC329/1  "<C_Opti_Speed_Slope>"
  BusSelector/74 -> DTC303/1  "<C_Gain_Press_Max>"
  BusSelector/51 -> DTC280/1  "<C_BCS_Flight_Speed_Min>"
  DTC291/1 -> Out62/1
  DTC314/1 -> Out85/1
  BusSelector/22 -> DTC251/1  "<CT_LandingSpunUpConf>"
  BusSelector/34 -> DTC263/1  "<C_Adher_Opt_Slope>"
  BusSelector/50 -> DTC279/1  "<C_BCS_Dflt_Accel4>"
  BusSelector/82 -> DTC311/1  "<C_I_AS_PB_OW_Thr_Auth>"
  DTC293/1 -> Out64/1
  BusSelector/117 -> DTC346/1  "<C_Slip_Max_BSL_WD>"
  BusSelector/4 -> DTC233/1  "<CT_Conf_BCS_Accel2_Fail>"
  BusSelector/9 -> DTC238/1  "<CT_Conf_BSL_WD_Mon_SL>"
  DTC320/1 -> Out91/1
  BusSelector/67 -> DTC296/1  "<C_Delta_Target_Speed>"
  DTC265/1 -> Out36/1
  BusSelector/48 -> DTC277/1  "<C_BCS_Coeff_Mult_Inf_Ref>"
  BusSelector/112 -> DTC341/1  "<C_SV_P_To_I_Slope>"
  BusSelector/12 -> DTC241/1  "<CT_Conf_Max_Duration_Phase2>"
  BusSelector/75 -> DTC304/1  "<C_Gain_Press_Min>"
  BusSelector/72 -> DTC301/1  "<C_FilloutPressureMargin>"
  DTC332/1 -> Out103/1
  BusSelector/115 -> DTC344/1  "<C_Slip_Coef_BKLoss>"
  BusSelector/17 -> DTC246/1  "<CT_Conf_No_BSL_WD>"
  DTC287/1 -> Out58/1
  BusSelector/15 -> DTC244/1  "<CT_Conf_No_BGam_Step>"
  DTC280/1 -> Out51/1
  BusSelector/62 -> DTC291/1  "<C_Dec_TG_Gam_Max>"
  DTC230/1 -> Out1/1
  DTC341/1 -> Out112/1
  BusSelector/14 -> DTC243/1  "<CT_Conf_Nlg_Ground_nominal>"
  BusSelector/68 -> DTC297/1  "<C_DenAccu_BSL_Max>"
  BusSelector/135 -> DTC364/1  "<C_TG_Gam_Min_Offset>"
  BusSelector/61 -> DTC290/1  "<C_Coef_TG_Gam_Min>"
  BusSelector/87 -> DTC316/1  "<C_Inv_Gain_Stat_AS>"
  BusSelector/106 -> DTC335/1  "<C_P_Com_Thr_BKLoss>"
  BusSelector/10 -> DTC239/1  "<CT_Conf_BrakeFillingTimeout>"
  BusSelector/140 -> DTC369/1  "<C_TakeOffAccel_Thr>"
  BusSelector/96 -> DTC325/1  "<C_Opti_Speed_Coef>"
  BusSelector/60 -> DTC289/1  "<C_BrakingOrderedMargin>"
  BusSelector/20 -> DTC249/1  "<CT_Filt_PT_Filt_Autom>"
  DTC308/1 -> Out79/1
  DTC355/1 -> Out126/1
  DTC316/1 -> Out87/1
  BusSelector/24 -> DTC253/1  "<C_Acc_BKLoss_Offset>"
  DTC317/1 -> Out88/1
  DTC309/1 -> Out80/1
  BusSelector/52 -> DTC281/1  "<C_BCS_Gbl_Ref_Speed_Init>"
  BusSelector/127 -> DTC356/1  "<C_Step_Size_Offset>"
  BusSelector/8 -> DTC237/1  "<CT_Conf_BSL_WD_Mon_FA>"
  DTC264/1 -> Out35/1
  DTC275/1 -> Out46/1
  DTC245/1 -> Out16/1
  DTC354/1 -> Out125/1
  DTC363/1 -> Out134/1
  DTC251/1 -> Out22/1
  DTC247/1 -> Out18/1
  DTC365/1 -> Out136/1
  DTC315/1 -> Out86/1
  DTC261/1 -> Out32/1
  DTC244/1 -> Out15/1
  DTC254/1 -> Out25/1
  DTC235/1 -> Out6/1
  DTC367/1 -> Out138/1
  DTC234/1 -> Out5/1
  DTC298/1 -> Out69/1
  DTC356/1 -> Out127/1
  DTC357/1 -> Out128/1
  DTC335/1 -> Out106/1
  DTC348/1 -> Out119/1
  DTC318/1 -> Out89/1
  DTC305/1 -> Out76/1
  DTC301/1 -> Out72/1
  DTC325/1 -> Out96/1
  DTC319/1 -> Out90/1
  DTC295/1 -> Out66/1
  DTC232/1 -> Out3/1
  DTC252/1 -> Out23/1
  DTC300/1 -> Out71/1
  DTC288/1 -> Out59/1
  DTC342/1 -> Out113/1
  DTC268/1 -> Out39/1
  DTC269/1 -> Out40/1
  DTC277/1 -> Out48/1
  DTC274/1 -> Out45/1
  DTC272/1 -> Out43/1
  DTC323/1 -> Out94/1
  DTC266/1 -> Out37/1
  DTC349/1 -> Out120/1
  DTC241/1 -> Out12/1
  DTC253/1 -> Out24/1
  DTC259/1 -> Out30/1
  DTC236/1 -> Out7/1
  DTC240/1 -> Out11/1
  DTC239/1 -> Out10/1
  DTC231/1 -> Out2/1
  DTC237/1 -> Out8/1
  DTC313/1 -> Out84/1
  DTC276/1 -> Out47/1
  DTC370/1 -> Out141/1
  DTC304/1 -> Out75/1
  DTC312/1 -> Out83/1
  DTC321/1 -> Out92/1
  DTC299/1 -> Out70/1
  DTC333/1 -> Out104/1
  DTC256/1 -> Out27/1
  DTC271/1 -> Out42/1
  DTC290/1 -> Out61/1
  DTC281/1 -> Out52/1
  DTC297/1 -> Out68/1
  DTC279/1 -> Out50/1
  DTC248/1 -> Out19/1
  In1/1 -> BusSelector/1
  DTC258/1 -> Out29/1
  DTC368/1 -> Out139/1
  DTC292/1 -> Out63/1
  DTC306/1 -> Out77/1
  DTC243/1 -> Out14/1
  DTC307/1 -> Out78/1
  DTC322/1 -> Out93/1
  DTC326/1 -> Out97/1
  DTC338/1 -> Out109/1
  DTC362/1 -> Out133/1
  DTC262/1 -> Out33/1
  DTC267/1 -> Out38/1
  DTC346/1 -> Out117/1
  DTC327/1 -> Out98/1
  DTC336/1 -> Out107/1
  DTC369/1 -> Out140/1
  DTC255/1 -> Out26/1
  DTC289/1 -> Out60/1
  DTC372/1 -> Out143/1
  DTC331/1 -> Out102/1
  DTC302/1 -> Out73/1
  DTC283/1 -> Out54/1
  DTC351/1 -> Out122/1
  DTC366/1 -> Out137/1
  DTC282/1 -> Out53/1
  DTC359/1 -> Out130/1
  DTC324/1 -> Out95/1

== system MATLAB_TEST/AVIONICS/Brake_Control_Module_Side_A/BCSA Controller CP/BCM_COM_PROC_P2_5/BCM_COM_PROC_P2_5/Subsystem ==
  In1 : Inport
  BusSelector : BusSelector  OutputSignals=CT_BCS_WS_First_Filter,C_BCS_AS_Perf_Gain,C_BCS_AS_Perf_Offset,C_BCS_I_AS_PB_Perf,C_BCS_P_Com_Perf,C_BCS_Tach_Speed_Init,C_BCS_Tach_Speed_Inval,C_BCS_WS_Noise_Factor,C_Filt_BCS_AS_Fast,C_Filt_BCS_AS_Perf_Max,C_Filt_BCS_AS_Perf_Min,C_Filt_BCS_AS_Slow,C_Tachometer_Min_Frequency,C_WST_OR_THR,C_Wheel_Speed_Conversion_Factor,C_Wheel_Speed_Default_Value,C_Wst_RateLim_Max,RateLim_Max,Tach_Speed_Init,Tach_Speed_Inval,WS_Noise_Factor,c_DCL_Law_CT_BCS_WS_First_Filter_Acc_AC,c_DCL_Law_CutOffFrequencyVSGRS_Law,c_DCL_Law_Strategie,c_DCL_Law_filt_8Hz
  DTC{12..34,36} (24 alike) : DataTypeConversion  OutDataTypeStr=single  SaturateOnIntegerOverflow=on  RndMeth=Zero
  DTC35 : DataTypeConversion  OutDataTypeStr=boolean  SaturateOnIntegerOverflow=on  RndMeth=Zero
  Out1 : Outport
  Out2 : Outport  Port=2
  Out3 : Outport  Port=3
  Out4 : Outport  Port=4
  Out5 : Outport  Port=5
  Out6 : Outport  Port=6
  Out7 : Outport  Port=7
  Out8 : Outport  Port=8
  Out9 : Outport  Port=9
  Out10 : Outport  Port=10
  Out11 : Outport  Port=11
  Out12 : Outport  Port=12
  Out13 : Outport  Port=13
  Out14 : Outport  Port=14
  Out15 : Outport  Port=15
  Out16 : Outport  Port=16
  Out17 : Outport  Port=17
  Out18 : Outport  Port=18
  Out19 : Outport  Port=19
  Out20 : Outport  Port=20
  Out21 : Outport  Port=21
  Out22 : Outport  Port=22
  Out23 : Outport  Port=23
  Out24 : Outport  Port=24
  Out25 : Outport  Port=25
  wires:
  BusSelector/5 -> DTC16/1  "<C_BCS_P_Com_Perf>"
  BusSelector/8 -> DTC19/1  "<C_BCS_WS_Noise_Factor>"
  DTC15/1 -> Out4/1
  BusSelector/13 -> DTC24/1  "<C_Tachometer_Min_Frequency>"
  DTC27/1 -> Out16/1
  DTC14/1 -> Out3/1
  BusSelector/1 -> DTC12/1  "<CT_BCS_WS_First_Filter>"
  DTC21/1 -> Out10/1
  BusSelector/6 -> DTC17/1  "<C_BCS_Tach_Speed_Init>"
  BusSelector/20 -> DTC31/1  "<Tach_Speed_Inval>"
  BusSelector/25 -> DTC36/1  "<c_DCL_Law_filt_8Hz>"
  BusSelector/15 -> DTC26/1  "<C_Wheel_Speed_Conversion_Factor>"
  BusSelector/12 -> DTC23/1  "<C_Filt_BCS_AS_Slow>"
  DTC13/1 -> Out2/1
  BusSelector/7 -> DTC18/1  "<C_BCS_Tach_Speed_Inval>"
  DTC18/1 -> Out7/1
  BusSelector/10 -> DTC21/1  "<C_Filt_BCS_AS_Perf_Max>"
  BusSelector/18 -> DTC29/1  "<RateLim_Max>"
  DTC33/1 -> Out22/1
  BusSelector/4 -> DTC15/1  "<C_BCS_I_AS_PB_Perf>"
  DTC20/1 -> Out9/1
  BusSelector/16 -> DTC27/1  "<C_Wheel_Speed_Default_Value>"
  DTC25/1 -> Out14/1
  BusSelector/11 -> DTC22/1  "<C_Filt_BCS_AS_Perf_Min>"
  BusSelector/17 -> DTC28/1  "<C_Wst_RateLim_Max>"
  BusSelector/21 -> DTC32/1  "<WS_Noise_Factor>"
  DTC12/1 -> Out1/1
  BusSelector/14 -> DTC25/1  "<C_WST_OR_THR>"
  DTC31/1 -> Out20/1
  BusSelector/23 -> DTC34/1  "<c_DCL_Law_CutOffFrequencyVSGRS_Law>"
  BusSelector/9 -> DTC20/1  "<C_Filt_BCS_AS_Fast>"
  BusSelector/19 -> DTC30/1  "<Tach_Speed_Init>"
  BusSelector/22 -> DTC33/1  "<c_DCL_Law_CT_BCS_WS_First_Filter_Acc_AC>"
  BusSelector/24 -> DTC35/1  "<c_DCL_Law_Strategie>"
  BusSelector/3 -> DTC14/1  "<C_BCS_AS_Perf_Offset>"
  DTC30/1 -> Out19/1
  DTC17/1 -> Out6/1
  BusSelector/2 -> DTC13/1  "<C_BCS_AS_Perf_Gain>"
  DTC19/1 -> Out8/1
  DTC35/1 -> Out24/1
  DTC23/1 -> Out12/1
  DTC34/1 -> Out23/1
  DTC29/1 -> Out18/1
  DTC32/1 -> Out21/1
  DTC26/1 -> Out15/1
  DTC36/1 -> Out25/1
  DTC24/1 -> Out13/1
  DTC16/1 -> Out5/1
  DTC28/1 -> Out17/1
  DTC22/1 -> Out11/1
  In1/1 -> BusSelector/1
